simulink model "seat_heating_control"  (R2020a)
settings: Solver=FixedStepDiscrete  StartTime=0.0  StopTime=10.0  FixedStep=0.01  RelTol=1e-3
undefined symbols (not defined in the file or in its folder): HeatingActivate_SetHeatingCoil, IDT_PowerState, RTE_OK, temp, TemperatureRanges_TemperatureStage1, TemperatureRanges_TemperatureStage2, TemperatureRanges_TemperatureStage3
settings Model: Creator=nabilekhoury  LastModifiedBy=yatishc
settings DataIOCC: SaveFormat=StructureWithTime
settings OptimizationCC: DefaultParameterBehavior=Inlined  EnhancedBackFolding=on  PassReuseOutputArgsAs=Individual arguments  ZeroExternalMemoryAtStartup=off  ZeroInternalMemoryAtStartup=off  OptimizeBlockOrder=speed  DifferentSizesBufferReuse=on  OptimizationCustomize=off  EfficientTunableParamExpr=on
settings DebuggingCC: ParameterTunabilityLossMsg=error  ArithmeticOperatorsInVariantConditions=warning
settings ModelReferenceCC: ModelReferenceNumInstancesAllowed=Single
settings SFSimCC: MATLABDynamicMemAlloc=off  CustomCodeUndefinedFunction=UseInterfaceOnly
settings RTWCC: Description=AUTOSAR  SystemTargetFile=autosar.tlc  GenCodeOnly=on  TemplateMakefile=ert_default_tmf  GenerateReport=on  IncludeHyperlinkInReport=on  LaunchReport=on  GenerateTraceInfo=on  GenerateTraceReport=on  GenerateTraceReportSl=on  GenerateTraceReportSf=on  GenerateTraceReportEml=on
settings CodeAppCC: ForceParamTrailComments=on  IgnoreCustomStorageClasses=off  OperatorAnnotations=on  SimulinkDataObjDesc=on  SFDataObjDesc=on  InsertBlockDesc=on
settings STFCustomTargetCC: TargetLangStandard=C99 (ISO)  MultiwordLength=256  ParMdlRefBuildCompliant=on  CompOptLevelCompliant=on  IncludeMdlTerminateFcn=off  CombineOutputUpdateFcns=on  SuppressErrorStatus=on  ERTCustomFileBanners=on  SupportNonFinite=off  SupportComplex=off  SupportContinuousTime=off  SupportNonInlinedSFcns=off  RemoveResetFunc=on  MATLABClassNameForMDSCustomization=Simulink.SoftwareTarget.ERTCustomization  AutosarCompliant=on  UseToolchainInfoCompliant=on  LookupTableObjectStructAxisOrder=2,1,3,4,...  LUTObjectStructOrderEvenSpacing=Size,Table,Breakpoints  SystemTargetFile=autosar.tlc
settings ERTTargetCC: TargetLangStandard=C99 (ISO)  ConcurrentExecutionCompliant=off  IncludeMdlTerminateFcn=off  SuppressErrorStatus=on  SupportNonFinite=off  SupportComplex=off  ModelStepFunctionPrototypeControlCompliant=off  CPPClassGenCompliant=off  AutosarCompliant=on  LookupTableObjectStructAxisOrder=2,1,3,4,...  LUTObjectStructOrderEvenSpacing=Size,Table,Breakpoints  InlinedParameterPlacement=NonHierarchical  ERTCustomFileTemplate=example_file_process.tlc

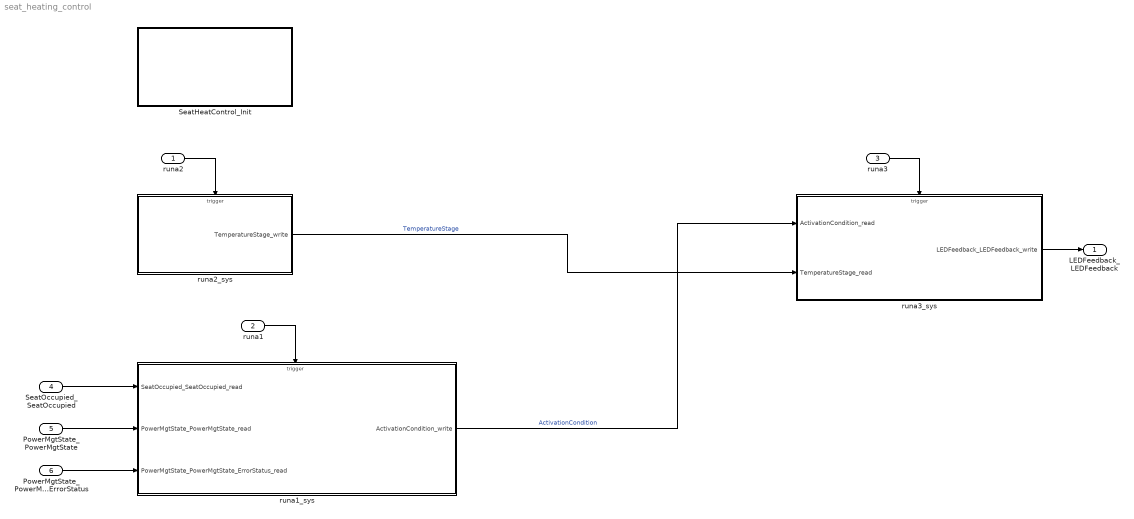
== system seat_heating_control ==
  runa2 : Inport  SampleTime=0.01  OutputFunctionCall=on
  runa1 : Inport  Port=2  SampleTime=0.01  OutputFunctionCall=on
  runa3 : Inport  Port=3  SampleTime=0.01  OutputFunctionCall=on
  SeatOccupied_SeatOccupied : Inport  Port=4  OutDataTypeStr=IDT_SeatStatus  PortDimensions=1
  PowerMgtState_PowerMgtState : Inport  Port=5  OutDataTypeStr=Enum: IDT_PowerState  PortDimensions=1
  PowerMgtState_PowerMgtState_ErrorStatus : Inport  Port=6  OutDataTypeStr=uint8  PortDimensions=1
  SeatHeatControl_Init : Subsystem
  runa1_sys : Subsystem
  runa2_sys : Subsystem
  runa3_sys : Subsystem
  LEDFeedback_LEDFeedback : Outport  OutDataTypeStr=boolean  PortDimensions=3
  wires:
  SeatOccupied_SeatOccupied/1 -> runa1_sys/1(SeatOccupied_SeatOccupied_read)
  PowerMgtState_PowerMgtState/1 -> runa1_sys/2(PowerMgtState_PowerMgtState_read)
  PowerMgtState_PowerMgtState_ErrorStatus/1 -> runa1_sys/3(PowerMgtState_PowerMgtState_ErrorStatus_read)
  runa3_sys/1(LEDFeedback_LEDFeedback_write) -> LEDFeedback_LEDFeedback/1
  runa2_sys/1(TemperatureStage_write) -> runa3_sys/2(TemperatureStage_read)  "TemperatureStage"
  runa1_sys/1(ActivationCondition_write) -> runa3_sys/1(ActivationCondition_read)  "ActivationCondition"
  runa2/1 -> runa2_sys/Trigger
  runa1/1 -> runa1_sys/Trigger
  runa3/1 -> runa3_sys/Trigger

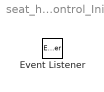
== system seat_heating_control/SeatHeatControl_Init ==
  Event Listener : EventListener  EventName=reset

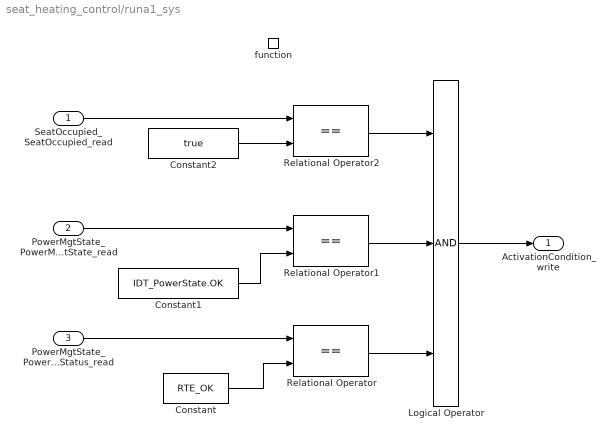
== system seat_heating_control/runa1_sys ==
  SeatOccupied_SeatOccupied_read : Inport
  PowerMgtState_PowerMgtState_read : Inport  Port=2
  PowerMgtState_PowerMgtState_ErrorStatus_read : Inport  Port=3
  function : TriggerPort  TriggerType=function-call  VariantControl=(inherit)  SampleTimeType=periodic  SampleTime=-1
  Constant : Constant  Value=RTE_OK
  Constant1 : Constant  Value=IDT_PowerState.OK
  Constant2 : Constant  Value=true
  Logical Operator : Logic  Inputs=3  AllPortsSameDT=off  OutDataTypeStr=boolean
  Relational Operator : RelationalOperator  Operator===  OutDataTypeStr=boolean  RndMeth=Simplest
  Relational Operator1 : RelationalOperator  Operator===  OutDataTypeStr=boolean  RndMeth=Simplest
  Relational Operator2 : RelationalOperator  Operator===  OutDataTypeStr=boolean  RndMeth=Simplest
  ActivationCondition_write : Outport  OutDataTypeStr=boolean  PortDimensions=1  InitialOutput=0
  wires:
  Logical Operator/1 -> ActivationCondition_write/1
  PowerMgtState_PowerMgtState_ErrorStatus_read/1 -> Relational Operator/1
  PowerMgtState_PowerMgtState_read/1 -> Relational Operator1/1
  Constant2/1 -> Relational Operator2/2
  SeatOccupied_SeatOccupied_read/1 -> Relational Operator2/1
  Relational Operator2/1 -> Logical Operator/1
  Constant1/1 -> Relational Operator1/2
  Relational Operator/1 -> Logical Operator/3
  Relational Operator1/1 -> Logical Operator/2
  Constant/1 -> Relational Operator/2

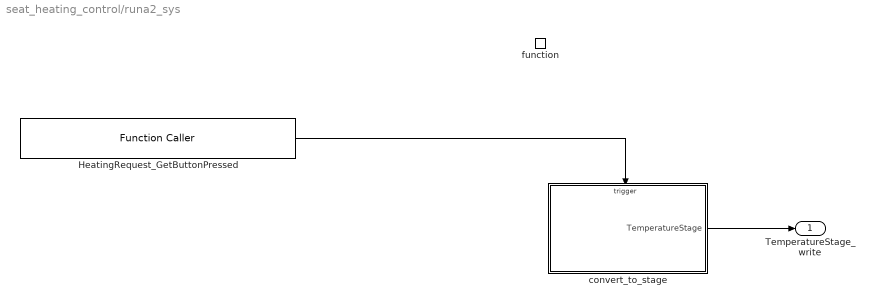
== system seat_heating_control/runa2_sys ==
  function : TriggerPort  TriggerType=function-call  VariantControl=(inherit)  SampleTimeType=periodic  SampleTime=-1
  HeatingRequest_GetButtonPressed : FunctionCaller  FunctionPrototype=status = HeatingRequest_GetButtonPressed()  OutputArgumentSpecifications=P_IDT_ButtonStatus
  convert_to_stage : Subsystem
  TemperatureStage_write : Outport  OutDataTypeStr=uint8  PortDimensions=1  InitialOutput=0
  wires:
  convert_to_stage/1(TemperatureStage) -> TemperatureStage_write/1
  HeatingRequest_GetButtonPressed/1 -> convert_to_stage/Trigger

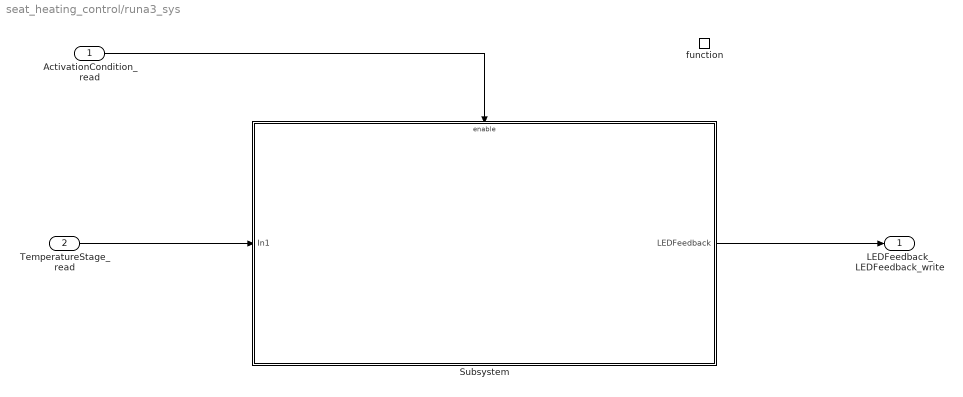
== system seat_heating_control/runa3_sys ==
  ActivationCondition_read : Inport
  TemperatureStage_read : Inport  Port=2
  function : TriggerPort  TriggerType=function-call  VariantControl=(inherit)  SampleTimeType=periodic  SampleTime=-1
  Subsystem : Subsystem
  LEDFeedback_LEDFeedback_write : Outport
      settings: EnsureOutportIsVirtual=on
  wires:
  ActivationCondition_read/1 -> Subsystem/Enable
  TemperatureStage_read/1 -> Subsystem/1(In1)
  Subsystem/1(LEDFeedback) -> LEDFeedback_LEDFeedback_write/1

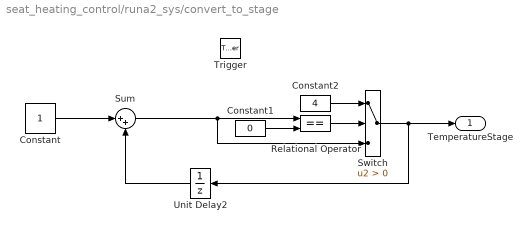
== system seat_heating_control/runa2_sys/convert_to_stage ==
  Trigger : TriggerPort  VariantControl=Variant  PortDimensions=1
  Constant : Constant  OutDataTypeStr=Inherit: Inherit via back propagation
  Constant1 : Constant  Value=0  OutDataTypeStr=Inherit: Inherit via back propagation
  Constant2 : Constant  Value=4  OutDataTypeStr=Inherit: Inherit via back propagation
  Relational Operator : RelationalOperator  Operator===  OutDataTypeStr=boolean  RndMeth=Simplest
  Sum : Sum  Inputs=|++
  Switch : Switch  Criteria=u2 > Threshold
  Unit Delay2 : UnitDelay  SampleTime=-1  HasFrameUpgradeWarning=on
      settings: AttributesFormatString=Init = %<InitialCondition>
  TemperatureStage : Outport  InitialOutput=0
  wires:
  Switch/1 -> TemperatureStage/1, Unit Delay2/1
  Constant2/1 -> Switch/1
  Unit Delay2/1 -> Sum/2
  Constant1/1 -> Relational Operator/2
  Sum/1 -> Switch/3, Relational Operator/1
  Constant/1 -> Sum/1
  Relational Operator/1 -> Switch/2

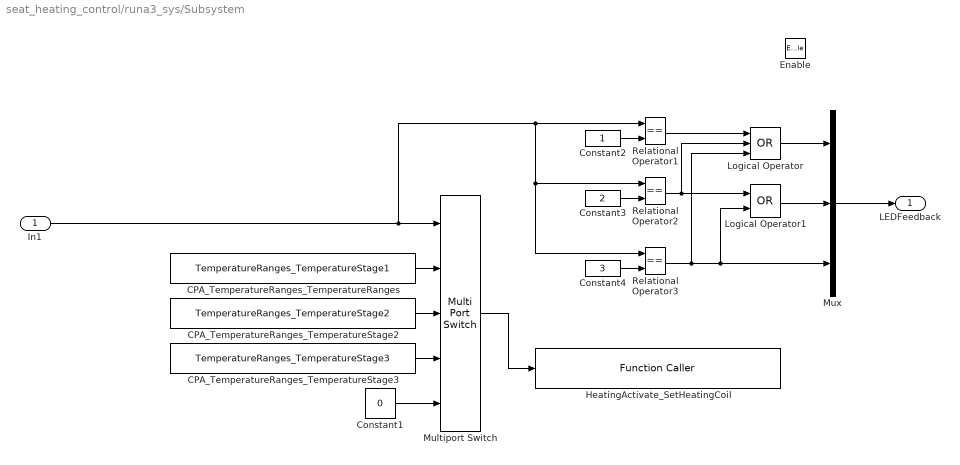
== system seat_heating_control/runa3_sys/Subsystem ==
  In1 : Inport
  Enable : EnablePort
  CPA_TemperatureRanges_TemperatureRanges : Constant  Value=TemperatureRanges_TemperatureStage1
  CPA_TemperatureRanges_TemperatureStage2 : Constant  Value=TemperatureRanges_TemperatureStage2
  CPA_TemperatureRanges_TemperatureStage3 : Constant  Value=TemperatureRanges_TemperatureStage3
  Constant1 : Constant  Value=0
  Constant2 : Constant  OutDataTypeStr=Inherit: Inherit via back propagation
  Constant3 : Constant  Value=2  OutDataTypeStr=Inherit: Inherit via back propagation
  Constant4 : Constant  Value=3  OutDataTypeStr=Inherit: Inherit via back propagation
  HeatingActivate_SetHeatingCoil : FunctionCaller  FunctionPrototype=HeatingActivate_SetHeatingCoil(temp)  InputArgumentSpecifications=P_IDT_Temperature
  Logical Operator : Logic  Operator=OR  Inputs=3  AllPortsSameDT=off  OutDataTypeStr=boolean
  Logical Operator1 : Logic  Operator=OR  AllPortsSameDT=off  OutDataTypeStr=boolean
  Multiport Switch : MultiPortSwitch  DataPortIndices={0,1,2,3}  DataPortForDefault=Additional data port  DiagnosticForDefault=None  OutDataTypeStr=IDT_Temperature
  Mux : Mux  Inputs=3
  Relational Operator1 : RelationalOperator  Operator===  OutDataTypeStr=boolean  RndMeth=Simplest
  Relational Operator2 : RelationalOperator  Operator===  OutDataTypeStr=boolean  RndMeth=Simplest
  Relational Operator3 : RelationalOperator  Operator===  OutDataTypeStr=boolean  RndMeth=Simplest
  LEDFeedback : Outport
  wires:
  In1/1 -> Relational Operator3/1, Relational Operator2/1, Relational Operator1/1, Multiport Switch/1
  Constant2/1 -> Relational Operator1/2
  Constant4/1 -> Relational Operator3/2
  Mux/1 -> LEDFeedback/1
  CPA_TemperatureRanges_TemperatureStage2/1 -> Multiport Switch/3
  Relational Operator2/1 -> Logical Operator1/1, Logical Operator/2
  Relational Operator1/1 -> Logical Operator/1
  Constant3/1 -> Relational Operator2/2
  Relational Operator3/1 -> Logical Operator/3, Logical Operator1/2, Mux/3
  Multiport Switch/1 -> HeatingActivate_SetHeatingCoil/1
  Constant1/1 -> Multiport Switch/5
  CPA_TemperatureRanges_TemperatureStage3/1 -> Multiport Switch/4
  CPA_TemperatureRanges_TemperatureRanges/1 -> Multiport Switch/2
  Logical Operator/1 -> Mux/1
  Logical Operator1/1 -> Mux/2
